simulink model "HDL_Genratable_DUMMY_Subsystem"  (R2019a)
settings: Solver=FixedStepDiscrete  StartTime=0.0  StopTime=stop_time  RelTol=1e-3
InitFcn:
  | sm_callback_init
StopFcn:
  | sm_callback_stop
undefined symbols (not defined in the file or in its folder): mp
libraries: simulink x4
settings Model: Creator=Ross  LastModifiedBy=justin
settings DataIOCC: SaveOutput=off  SaveTime=off  ReturnWorkspaceOutputs=off
settings OptimizationCC: BlockReduction=off  ConditionallyExecuteInputs=off  DefaultParameterBehavior=Inlined
settings DebuggingCC: ReadBeforeWriteMsg=DisableAll  WriteAfterWriteMsg=DisableAll  WriteAfterReadMsg=DisableAll  AlgebraicLoopMsg=error  MultiTaskDSMMsg=none  SingleTaskRateTransMsg=error  PregeneratedLibrarySubsystemCodeDiagnostic=none  ArithmeticOperatorsInVariantConditions=warning
settings HardwareCC: ProdBitPerPointer=32  ProdBitPerSizeT=32  ProdBitPerPtrDiffT=32  ProdLargestAtomicFloat=None  ProdIntDivRoundTo=Undefined  ProdEndianess=Unspecified  ProdWordSize=32  ProdHWDeviceType=ASIC/FPGA->ASIC/FPGA  TargetBitPerLong=64  TargetBitPerPointer=64  TargetBitPerSizeT=64  TargetBitPerPtrDiffT=64  TargetLongLongMode=on  TargetIntDivRoundTo=Zero  TargetEndianess=LittleEndian  TargetWordSize=64  TargetHWDeviceType=Custom Processor->MATLAB Host Computer  ProdEqTarget=off
settings ModelReferenceCC: UpdateModelReferenceTargets=IfOutOfDate
settings SFSimCC: SFSimEcho=off  SimUseLocalCustomCode=off
settings RTWCC: RTWUseLocalCustomCode=off

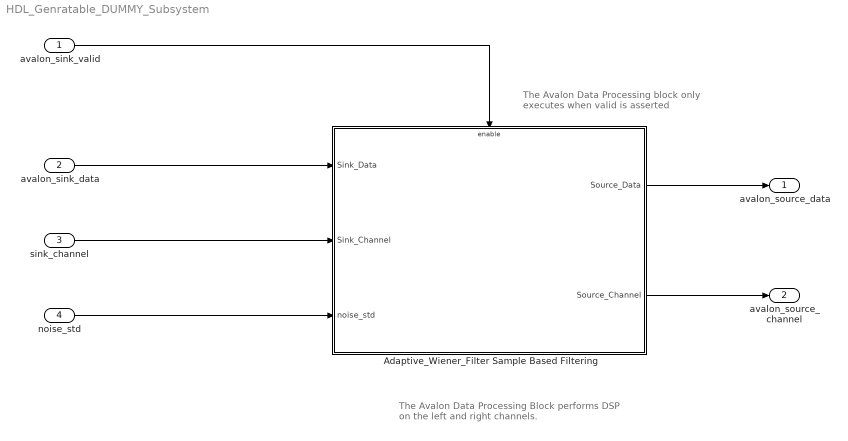
== system HDL_Genratable_DUMMY_Subsystem ==
  note: The Avalon Data Processing Block
      | performs DSP on the left and right channels.
  note: The Avalon Data Processing block
      | only executes when valid is asserted
  avalon_sink_valid : Inport  OutDataTypeStr=boolean  PortDimensions=[1 1]  SampleTime=[2.6041666666666666e-06,0]
  avalon_sink_data : Inport  Port=2  OutDataTypeStr=fixdt(1,32,28)  PortDimensions=[1 1]  SampleTime=[2.6041666666666666e-06,0]
  sink_channel : Inport  Port=3  OutDataTypeStr=fixdt(0,2,0)  PortDimensions=[1 1]  SampleTime=[2.6041666666666666e-06,0]
  noise_std : Inport  Port=4  OutDataTypeStr=fixdt(1,32,28)  PortDimensions=1  SampleTime=[2.6041666666666666e-06,0]
  Adaptive_Wiener_Filter Sample Based Filtering : Subsystem
  avalon_source_data : Outport  OutDataTypeStr=fixdt(1,32,28)  PortDimensions=[1 1]  SampleTime=[2.6041666666666666e-06,0]
  avalon_source_channel : Outport  Port=2  OutDataTypeStr=fixdt(0,2,0)  PortDimensions=[1 1]  SampleTime=[2.6041666666666666e-06,0]
  wires:
  Adaptive_Wiener_Filter Sample Based Filtering/2(Source_Channel) -> avalon_source_channel/1
  avalon_sink_valid/1 -> Adaptive_Wiener_Filter Sample Based Filtering/Enable
  avalon_sink_data/1 -> Adaptive_Wiener_Filter Sample Based Filtering/1(Sink_Data)
  sink_channel/1 -> Adaptive_Wiener_Filter Sample Based Filtering/2(Sink_Channel)
  Adaptive_Wiener_Filter Sample Based Filtering/1(Source_Data) -> avalon_source_data/1
  noise_std/1 -> Adaptive_Wiener_Filter Sample Based Filtering/3(noise_std)

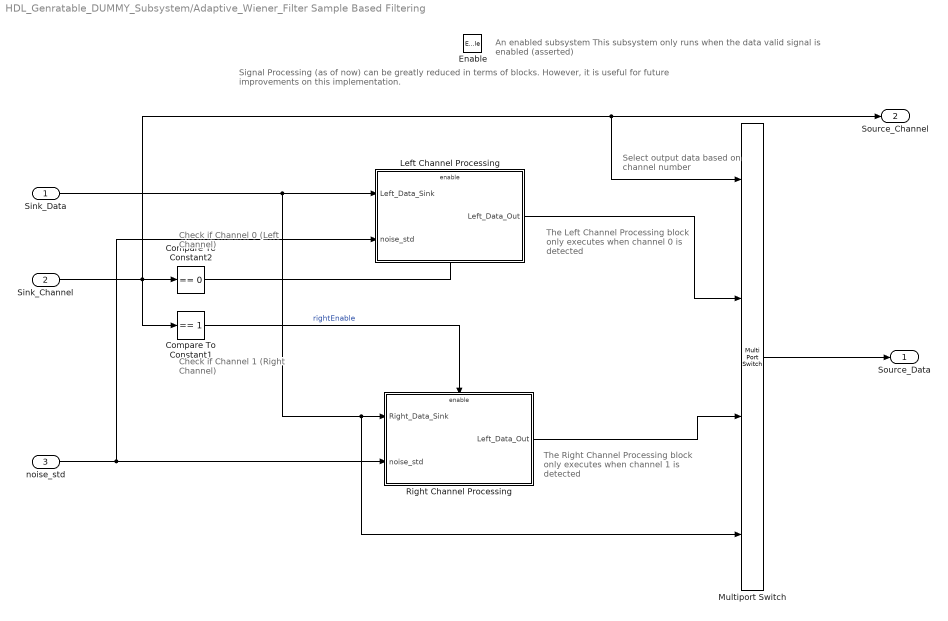
== system HDL_Genratable_DUMMY_Subsystem/Adaptive_Wiener_Filter Sample Based Filtering ==
  note: Check if Channel 1
      | (Right Channel)
  note: An enabled subsystem
      | This subsystem only runs when the data valid signal is enabled (asserted)
  note: Select output data
      | based on channel number
  note: Check if Channel 0
      | (Left Channel)
  note: The Right Channel Processing block
      | only executes when channel 1
      | is detected
  note: The Left Channel Processing block
      | only executes when channel 0
      | is detected
  note: Signal Processing (as of now) can be greatly reduced in terms of blocks.
      | However, it is useful for future improvements on this implementation.
  Sink_Data : Inport
  Sink_Channel : Inport  Port=2
  noise_std : Inport  Port=3
  Enable : EnablePort
  Compare To Constant1 : simulink/Logic and Bit Operations/Compare To Constant  relop===  const=1  OutDataTypeStr=boolean
  Compare To Constant2 : simulink/Logic and Bit Operations/Compare To Constant  relop===  const=0  OutDataTypeStr=boolean
  Left Channel Processing : Subsystem  TreatAsAtomicUnit=on
  Multiport Switch : MultiPortSwitch  DataPortOrder=Zero-based contiguous  zeroidx=on
  Right Channel Processing : Subsystem  TreatAsAtomicUnit=on
  Source_Data : Outport  InitialOutput=0
  Source_Channel : Outport  Port=2  InitialOutput=0
  wires:
  noise_std/1 -> Left Channel Processing/2(noise_std), Right Channel Processing/2(noise_std)
  Compare To Constant1/1 -> Right Channel Processing/Enable  "rightEnable"
  Sink_Channel/1 -> Compare To Constant2/1, Compare To Constant1/1, Multiport Switch/1, Source_Channel/1
  Right Channel Processing/1("Left_Data_Out ") -> Multiport Switch/3
  Sink_Data/1 -> Left Channel Processing/1(Left_Data_Sink), Multiport Switch/4, Right Channel Processing/1(Right_Data_Sink)
  Compare To Constant2/1 -> Left Channel Processing/Enable
  Multiport Switch/1 -> Source_Data/1
  Left Channel Processing/1("Left_Data_Out ") -> Multiport Switch/2

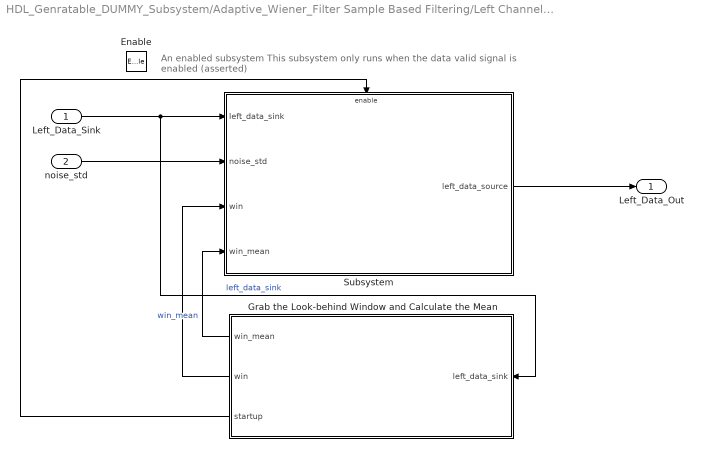
== system HDL_Genratable_DUMMY_Subsystem/Adaptive_Wiener_Filter Sample Based Filtering/Left Channel Processing ==
  note: An enabled subsystem
      | This subsystem only runs when the data valid signal is enabled (asserted)
  Left_Data_Sink : Inport
  noise_std : Inport  Port=2
  Enable : EnablePort
  Grab the Look-behind Window and Calculate the Mean : Subsystem
  Subsystem : Subsystem
  "Left_Data_Out " : Outport  InitialOutput=0
  wires:
  Grab the Look-behind Window and Calculate the Mean/3(startup) -> Subsystem/Enable
  Grab the Look-behind Window and Calculate the Mean/2(win) -> Subsystem/3(win)
  Grab the Look-behind Window and Calculate the Mean/1(win_mean) -> Subsystem/4(win_mean)  "win_mean"
  Subsystem/1(left_data_source) -> "Left_Data_Out "/1
  noise_std/1 -> Subsystem/2(noise_std)
  Left_Data_Sink/1 -> Subsystem/1(left_data_sink), Grab the Look-behind Window and Calculate the Mean/1(left_data_sink)  "left_data_sink"

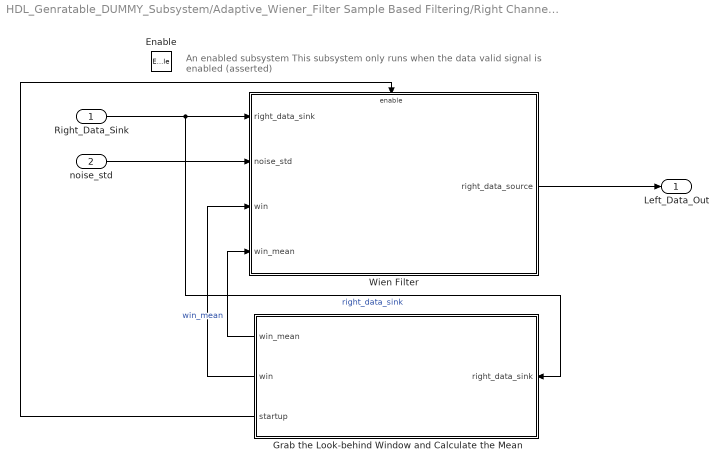
== system HDL_Genratable_DUMMY_Subsystem/Adaptive_Wiener_Filter Sample Based Filtering/Right Channel Processing ==
  note: An enabled subsystem
      | This subsystem only runs when the data valid signal is enabled (asserted)
  Right_Data_Sink : Inport
  noise_std : Inport  Port=2
  Enable : EnablePort
  Grab the Look-behind Window and Calculate the Mean : Subsystem
  Wien Filter : Subsystem
  "Left_Data_Out " : Outport  InitialOutput=0
  wires:
  Grab the Look-behind Window and Calculate the Mean/3(startup) -> Wien Filter/Enable
  Grab the Look-behind Window and Calculate the Mean/2(win) -> Wien Filter/3(win)
  Grab the Look-behind Window and Calculate the Mean/1(win_mean) -> Wien Filter/4(win_mean)  "win_mean"
  Wien Filter/1(right_data_source) -> "Left_Data_Out "/1
  noise_std/1 -> Wien Filter/2(noise_std)
  Right_Data_Sink/1 -> Wien Filter/1(right_data_sink), Grab the Look-behind Window and Calculate the Mean/1(right_data_sink)  "right_data_sink"

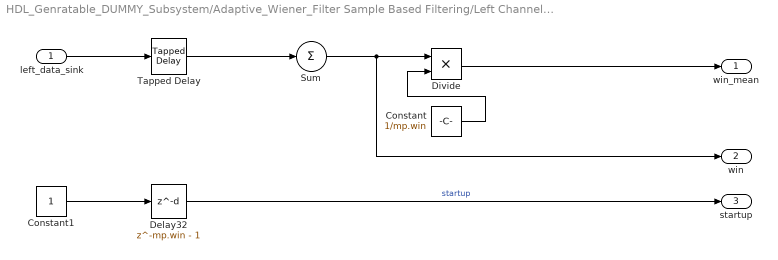
== system HDL_Genratable_DUMMY_Subsystem/Adaptive_Wiener_Filter Sample Based Filtering/Left Channel Processing/Grab the Look-behind Window and Calculate the Mean ==
  left_data_sink : Inport
  Constant : Constant  Value=1/mp.win  OutDataTypeStr=fixdt(1,mp.W_bits, mp.F_bits)  SampleTime=-1
  Constant1 : Constant  OutDataTypeStr=boolean  SampleTime=-1
  Delay32 : Delay  DelayLength=mp.win - 1
  Divide : Product  Inputs=**  OutDataTypeStr=Inherit: Same as first input
  Sum : Sum  Inputs=+  OutDataTypeStr=Inherit: Same as first input
  Tapped Delay : simulink/Discrete/Tapped Delay  vinit=0.0  samptime=-1  NumDelays=mp.win - 1  DelayOrder=Newest  includeCurrent=on
  win_mean : Outport  VectorParamsAs1DForOutWhenUnconnected=on
  win : Outport  Port=2  VectorParamsAs1DForOutWhenUnconnected=on
  startup : Outport  Port=3  VectorParamsAs1DForOutWhenUnconnected=on
  wires:
  Delay32/1 -> startup/1  "startup"
  Constant1/1 -> Delay32/1
  Divide/1 -> win_mean/1
  Constant/1 -> Divide/2
  Sum/1 -> Divide/1, win/1
  Tapped Delay/1 -> Sum/1
  left_data_sink/1 -> Tapped Delay/1

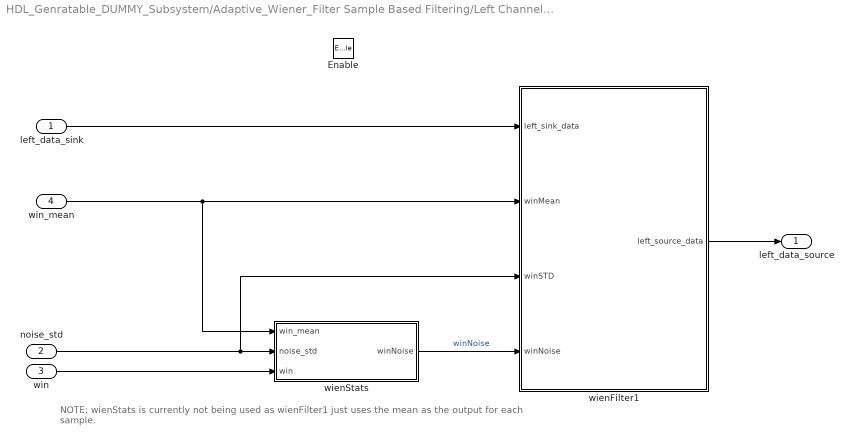
== system HDL_Genratable_DUMMY_Subsystem/Adaptive_Wiener_Filter Sample Based Filtering/Left Channel Processing/Subsystem ==
  note: NOTE: wienStats is currently not being used as wienFilter1 just uses the mean as the output for each sample.
  left_data_sink : Inport
  noise_std : Inport  Port=2
  win : Inport  Port=3
  win_mean : Inport  Port=4
  Enable : EnablePort
  wienFilter1 : Subsystem
  wienStats : Subsystem
  left_data_source : Outport  VectorParamsAs1DForOutWhenUnconnected=on
  wires:
  win/1 -> wienStats/3(win)
  left_data_sink/1 -> wienFilter1/1(left_sink_data)
  win_mean/1 -> wienStats/1(win_mean), wienFilter1/2(winMean)
  wienFilter1/1(left_source_data) -> left_data_source/1
  wienStats/1(winNoise) -> wienFilter1/4(winNoise)  "winNoise"
  noise_std/1 -> wienStats/2(noise_std), wienFilter1/3(winSTD)

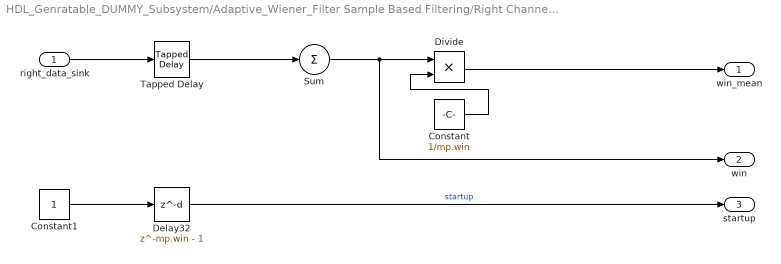
== system HDL_Genratable_DUMMY_Subsystem/Adaptive_Wiener_Filter Sample Based Filtering/Right Channel Processing/Grab the Look-behind Window and Calculate the Mean ==
  right_data_sink : Inport
  Constant : Constant  Value=1/mp.win  OutDataTypeStr=fixdt(1,mp.W_bits, mp.F_bits)  SampleTime=-1
  Constant1 : Constant  OutDataTypeStr=boolean  SampleTime=-1
  Delay32 : Delay  DelayLength=mp.win - 1
  Divide : Product  Inputs=**  OutDataTypeStr=Inherit: Same as first input
  Sum : Sum  Inputs=+  OutDataTypeStr=Inherit: Same as first input
  Tapped Delay : simulink/Discrete/Tapped Delay  vinit=0.0  samptime=-1  NumDelays=mp.win - 1  DelayOrder=Newest  includeCurrent=on
  win_mean : Outport  VectorParamsAs1DForOutWhenUnconnected=on
  win : Outport  Port=2  VectorParamsAs1DForOutWhenUnconnected=on
  startup : Outport  Port=3  VectorParamsAs1DForOutWhenUnconnected=on
  wires:
  Delay32/1 -> startup/1  "startup"
  Constant1/1 -> Delay32/1
  Divide/1 -> win_mean/1
  Constant/1 -> Divide/2
  Sum/1 -> Divide/1, win/1
  Tapped Delay/1 -> Sum/1
  right_data_sink/1 -> Tapped Delay/1

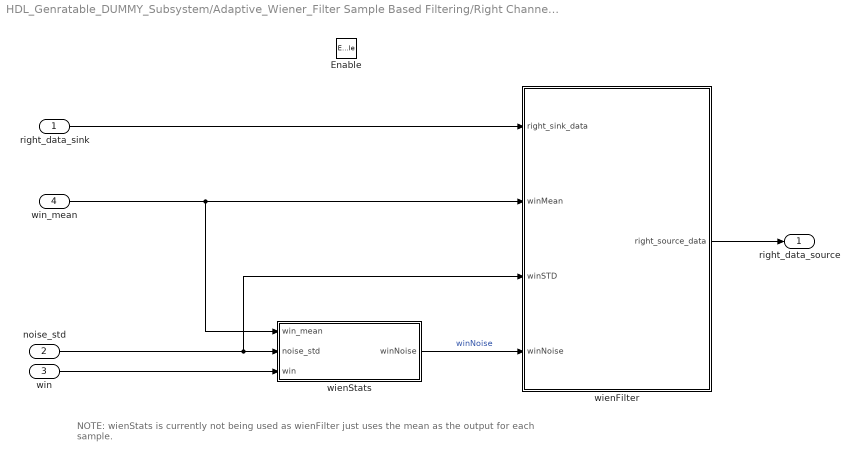
== system HDL_Genratable_DUMMY_Subsystem/Adaptive_Wiener_Filter Sample Based Filtering/Right Channel Processing/Wien Filter ==
  note: NOTE: wienStats is currently not being used as wienFilter just uses the mean as the output for each sample.
  right_data_sink : Inport
  noise_std : Inport  Port=2
  win : Inport  Port=3
  win_mean : Inport  Port=4
  Enable : EnablePort
  wienFilter : Subsystem
  wienStats : Subsystem
  right_data_source : Outport  VectorParamsAs1DForOutWhenUnconnected=on
  wires:
  win/1 -> wienStats/3(win)
  right_data_sink/1 -> wienFilter/1(right_sink_data)
  win_mean/1 -> wienStats/1(win_mean), wienFilter/2(winMean)
  wienFilter/1(right_source_data) -> right_data_source/1
  wienStats/1(winNoise) -> wienFilter/4(winNoise)  "winNoise"
  noise_std/1 -> wienStats/2(noise_std), wienFilter/3(winSTD)

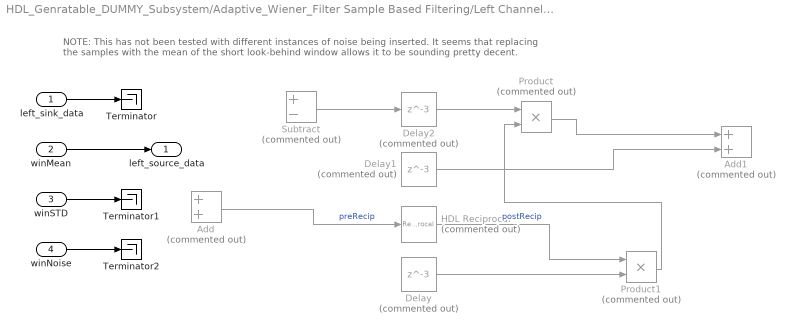
== system HDL_Genratable_DUMMY_Subsystem/Adaptive_Wiener_Filter Sample Based Filtering/Left Channel Processing/Subsystem/wienFilter1 ==
  note: NOTE: This has not been tested with different instances of noise being inserted.
      |
      | It seems that replacing the samples with the mean of the short look-behind window allows it to be sounding pretty decent.
  left_sink_data : Inport
  winMean : Inport  Port=2
  winSTD : Inport  Port=3
  winNoise : Inport  Port=4
  Add : Sum  Commented=on
  Add1 : Sum  Commented=on  OutDataTypeStr=Inherit: Same as first input
  Delay : Delay  Commented=on  DelayLength=3
  Delay1 : Delay  Commented=on  DelayLength=3
  Delay2 : Delay  Commented=on  DelayLength=3
  HDL Reciprocal : Reciprocal  Commented=on
  Product : Product  Commented=on  OutDataTypeStr=Inherit: Same as first input
  Product1 : Product  Commented=on  OutDataTypeStr=Inherit: Same as first input
  Subtract : Sum  Commented=on  Inputs=+-  OutDataTypeStr=Inherit: Same as first input
  Terminator : Terminator
  Terminator1 : Terminator
  Terminator2 : Terminator
  left_source_data : Outport  VectorParamsAs1DForOutWhenUnconnected=on
  wires:
  winMean/1 -> left_source_data/1
  winNoise/1 -> Terminator2/1
  winSTD/1 -> Terminator1/1
  Delay2/1 -> Product/1
  Product/1 -> Add1/1
  Delay1/1 -> Add1/2
  Delay/1 -> Product1/2
  Product1/1 -> Product/2
  HDL Reciprocal/1 -> Product1/1  "postRecip"
  Add/1 -> HDL Reciprocal/1  "preRecip"
  Subtract/1 -> Delay2/1
  left_sink_data/1 -> Terminator/1

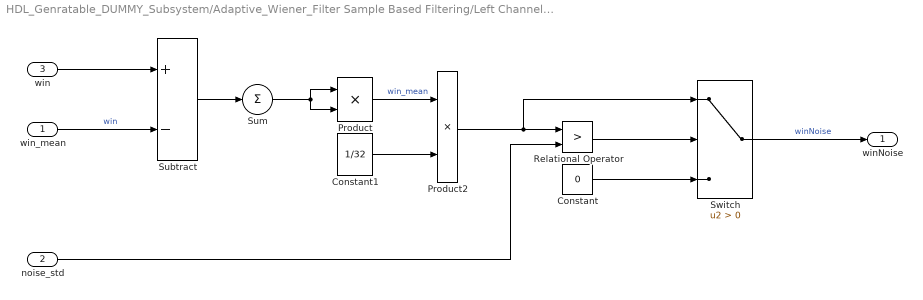
== system HDL_Genratable_DUMMY_Subsystem/Adaptive_Wiener_Filter Sample Based Filtering/Left Channel Processing/Subsystem/wienStats ==
  win_mean : Inport
  noise_std : Inport  Port=2
  win : Inport  Port=3
  Constant : Constant  Value=0  OutDataTypeStr=fixdt(1, mp.W_bits, mp.F_bits)  SampleTime=-1
  Constant1 : Constant  Value=1/32  OutDataTypeStr=fixdt(1,mp.W_bits,mp.F_bits)  SampleTime=-1
  Product : Product  OutDataTypeStr=fixdt(1, mp.W_bits+5, mp.F_bits)
  Product2 : Product  OutDataTypeStr=fixdt(1, mp.W_bits, mp.F_bits)
  Relational Operator : RelationalOperator  Operator=>  OutDataTypeStr=boolean  RndMeth=Nearest
  Subtract : Sum  Inputs=+-  OutDataTypeStr=Inherit: Same as first input
  Sum : Sum  Inputs=+  OutDataTypeStr=Inherit: Same as first input
  Switch : Switch  Criteria=u2 > Threshold
  winNoise : Outport  VectorParamsAs1DForOutWhenUnconnected=on
  wires:
  Constant/1 -> Switch/3
  Relational Operator/1 -> Switch/2
  Product2/1 -> Relational Operator/1, Switch/1
  noise_std/1 -> Relational Operator/2
  Product/1 -> Product2/1  "win_mean"
  Sum/1 -> Product/1, Product/2
  win_mean/1 -> Subtract/2  "win"
  win/1 -> Subtract/1
  Subtract/1 -> Sum/1
  Constant1/1 -> Product2/2
  Switch/1 -> winNoise/1  "winNoise"

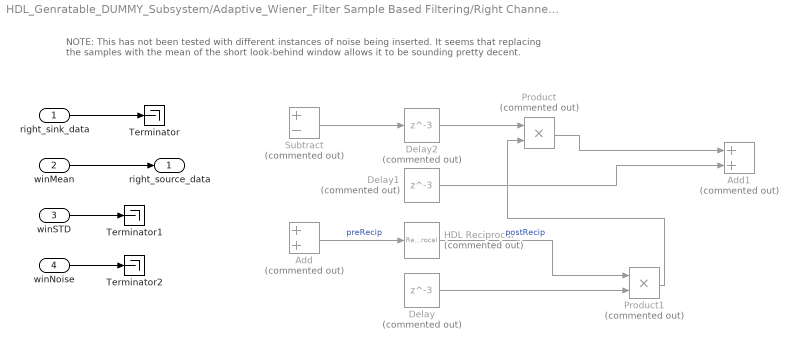
== system HDL_Genratable_DUMMY_Subsystem/Adaptive_Wiener_Filter Sample Based Filtering/Right Channel Processing/Wien Filter/wienFilter ==
  note: NOTE: This has not been tested with different instances of noise being inserted.
      |
      | It seems that replacing the samples with the mean of the short look-behind window allows it to be sounding pretty decent.
  right_sink_data : Inport
  winMean : Inport  Port=2
  winSTD : Inport  Port=3
  winNoise : Inport  Port=4
  Add : Sum  Commented=on
  Add1 : Sum  Commented=on  OutDataTypeStr=Inherit: Same as first input
  Delay : Delay  Commented=on  DelayLength=3
  Delay1 : Delay  Commented=on  DelayLength=3
  Delay2 : Delay  Commented=on  DelayLength=3
  HDL Reciprocal : Reciprocal  Commented=on
  Product : Product  Commented=on  OutDataTypeStr=Inherit: Same as first input
  Product1 : Product  Commented=on  OutDataTypeStr=Inherit: Same as first input
  Subtract : Sum  Commented=on  Inputs=+-  OutDataTypeStr=Inherit: Same as first input
  Terminator : Terminator
  Terminator1 : Terminator
  Terminator2 : Terminator
  right_source_data : Outport  VectorParamsAs1DForOutWhenUnconnected=on
  wires:
  winMean/1 -> right_source_data/1
  winNoise/1 -> Terminator2/1
  winSTD/1 -> Terminator1/1
  Delay2/1 -> Product/1
  Product/1 -> Add1/1
  Delay1/1 -> Add1/2
  Delay/1 -> Product1/2
  Product1/1 -> Product/2
  HDL Reciprocal/1 -> Product1/1  "postRecip"
  Add/1 -> HDL Reciprocal/1  "preRecip"
  Subtract/1 -> Delay2/1
  right_sink_data/1 -> Terminator/1

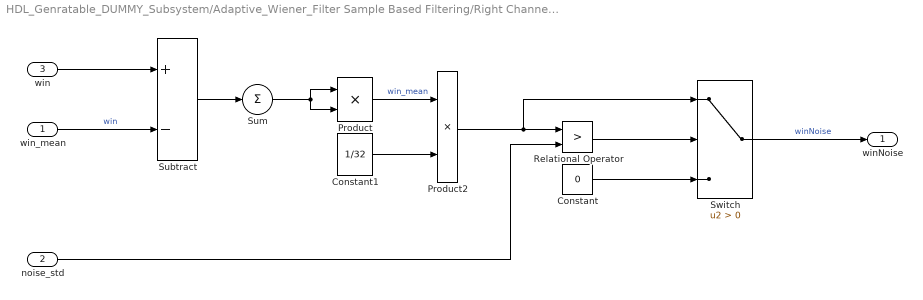
== system HDL_Genratable_DUMMY_Subsystem/Adaptive_Wiener_Filter Sample Based Filtering/Right Channel Processing/Wien Filter/wienStats ==
  win_mean : Inport
  noise_std : Inport  Port=2
  win : Inport  Port=3
  Constant : Constant  Value=0  OutDataTypeStr=fixdt(1, mp.W_bits, mp.F_bits)  SampleTime=-1
  Constant1 : Constant  Value=1/32  OutDataTypeStr=fixdt(1,mp.W_bits,mp.F_bits)  SampleTime=-1
  Product : Product  OutDataTypeStr=fixdt(1, mp.W_bits+5, mp.F_bits)
  Product2 : Product  OutDataTypeStr=fixdt(1, mp.W_bits, mp.F_bits)
  Relational Operator : RelationalOperator  Operator=>  OutDataTypeStr=boolean  RndMeth=Nearest
  Subtract : Sum  Inputs=+-  OutDataTypeStr=Inherit: Same as first input
  Sum : Sum  Inputs=+  OutDataTypeStr=Inherit: Same as first input
  Switch : Switch  Criteria=u2 > Threshold
  winNoise : Outport  VectorParamsAs1DForOutWhenUnconnected=on
  wires:
  Constant/1 -> Switch/3
  Relational Operator/1 -> Switch/2
  Product2/1 -> Relational Operator/1, Switch/1
  noise_std/1 -> Relational Operator/2
  Product/1 -> Product2/1  "win_mean"
  Sum/1 -> Product/1, Product/2
  win_mean/1 -> Subtract/2  "win"
  win/1 -> Subtract/1
  Subtract/1 -> Sum/1
  Constant1/1 -> Product2/2
  Switch/1 -> winNoise/1  "winNoise"
